simulink model "generator_of_imu"  (R2016b)
settings: Solver=ode8  StartTime=0.0  StopTime=500  FixedStep=0.01  RelTol=1e-3
undefined symbols (not defined in the file or in its folder): deg, rad, s
libraries: simulink x6, aerolibconvert2 x2, powerlib_meascontrol x2, aerolib6dof2 x1
settings Model: Creator=Utente  LastModifiedBy=Utente

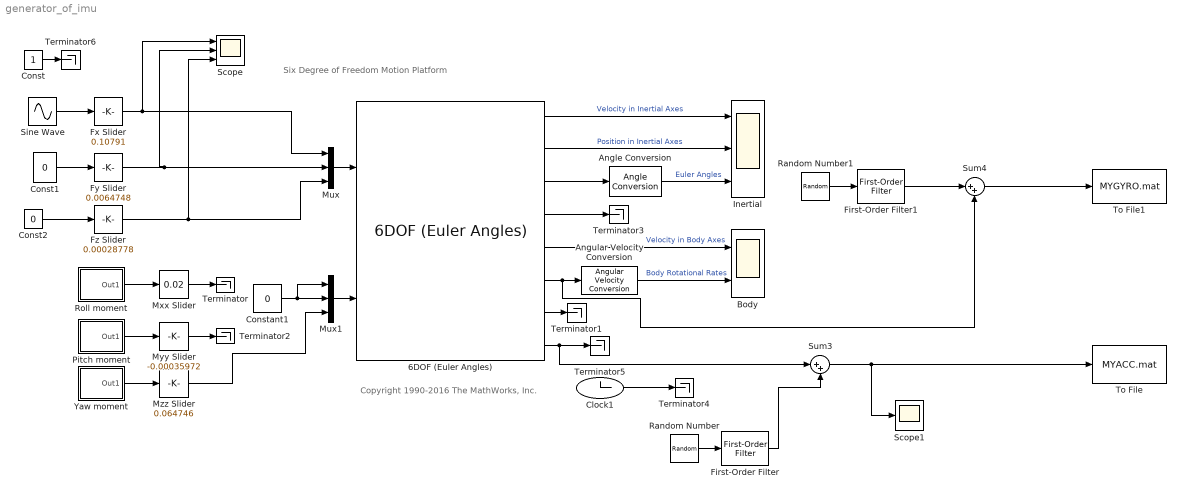
== system generator_of_imu ==
  note: Six Degree of Freedom Motion Platform
  note: Copyright 1990-2016 The MathWorks, Inc.
  6DOF (Euler Angles) : aerolib6dof2/6DOF (Euler Angles)  units=Metric (MKS)  mtype=Fixed  rep=Euler Angles  xme_0=[0 0 0]  Vm_0=[0 0 0]  eul_0=[0 0 0]  pm_0=[0 0 0]  mass_0=1.0  mass_e=0.5  mass_f=2.0  inertia=eye(3)  inertia_e=eye(3)  inertia_f=2*eye(3)  k_quat=1.0  vre_flag=on
  Angle Conversion : aerolibconvert2/Angle Conversion  IU=rad  OU=deg
  Angular Velocity Conversion : aerolibconvert2/Angular Velocity Conversion  IU=rad/s  OU=deg/s
  Body : Scope  NumInputPorts=2
  Clock1 : Clock
      settings: Decimation=100
  Const : Constant
  Const1 : Constant  Value=0
  Const2 : Constant  Value=0
  Constant1 : Constant  Value=0
  First-Order Filter : powerlib_meascontrol/Filters/First-Order Filter  FilterType=Lowpass  Tc=10  Ts=0.01  Initialize=on  Vac_Init=[0, 0, 60]  Vdc_Init=0  PlotResponse=off  FreqRange="[0,  200,  1]"
  First-Order Filter1 : powerlib_meascontrol/Filters/First-Order Filter  FilterType=Lowpass  Tc=50  Ts=0.01  Initialize=on  Vac_Init=[0, 0, 0]  Vdc_Init=0  PlotResponse=off  FreqRange="[0,  200,  1]"
  Fx Slider : simulink/Math Operations/Slider Gain  low=-1  gain=0.10791  high=1
  Fy Slider : simulink/Math Operations/Slider Gain  low=-1  gain=0.0064748  high=1
  Fz Slider : simulink/Math Operations/Slider Gain  low=-1  gain=0.00028778  high=1
  Inertial : Scope  NumInputPorts=3
  Mux : Mux  Inputs=3
  Mux1 : Mux  Inputs=3
  Mxx Slider : simulink/Math Operations/Slider Gain  low=0  gain=0.02  high=1
  Myy Slider : simulink/Math Operations/Slider Gain  low=-5  gain=-0.00035972  high=1
  Mzz Slider : simulink/Math Operations/Slider Gain  low=-3  gain=0.064746  high=3
  Pitch moment : Subsystem  mask(timed input){t=[0 3 3 4 4 5 5  7.5 7.5 8.5 8.5 9.5 9.5 10], u=[0 0  1 1 -1 -1.005 0 0 -1 -1 1 1 0 0]*3.138/2}
      mask prompts: t "time values:"; u "input values"
      mask Display: plot(t,u)
  Random Number : RandomNumber  Mean=[0;0;0]  Variance=0.09  SampleTime=0.01
  Random Number1 : RandomNumber  Mean=[0;0;0]  Variance=0.0140  SampleTime=0.01
  Roll moment : Subsystem  mask(timed input){t=[0 1 1 2 2  10], u=[1 1 -1 -.998  0 0]*3.144/2}
      mask prompts: t "time values:"; u "input values"
      mask Display: plot(t,u)
  Scope : Scope  NumInputPorts=3
  Scope1 : Scope
  Sine Wave : Sin  Amplitude=10  Frequency=10  SampleTime=0.1
  Sum3 : Sum  Inputs=|++
  Sum4 : Sum  Inputs=|++
  Terminator{,1..6} (7 alike) : Terminator
  To File : ToFile  Filename=MYACC.mat  SaveFormat=Timeseries
  To File1 : ToFile  Filename=MYGYRO.mat  SaveFormat=Timeseries
  Yaw moment : Subsystem  mask(timed input){t=[0 6 6 7 7 8 8 10], u=[0 0  -1 -1 1 1 1 1]*3.1/2}
      mask prompts: t "time values:"; u "input values"
      mask Display: plot(t,u)
  wires:
  Yaw moment/1(Out1) -> Mzz Slider/1
  Pitch moment/1(Out1) -> Myy Slider/1
  Roll moment/1(Out1) -> Mxx Slider/1
  Const2/1 -> Fz Slider/1
  Const1/1 -> Fy Slider/1
  Clock1/1 -> Terminator4/1
  Mux1/1 -> 6DOF (Euler Angles)/2
  Mzz Slider/1 -> Mux1/3
  Myy Slider/1 -> Terminator2/1
  Mxx Slider/1 -> Terminator/1
  Mux/1 -> 6DOF (Euler Angles)/1
  Fy Slider/1 -> Scope/2, Mux/2
  Fz Slider/1 -> Scope/3, Mux/3
  Fx Slider/1 -> Mux/1, Scope/1
  6DOF (Euler Angles)/4 -> Terminator3/1
  6DOF (Euler Angles)/7 -> Terminator1/1
  6DOF (Euler Angles)/3 -> Angle Conversion/1
  6DOF (Euler Angles)/5 -> Body/1  "Velocity in Body Axes"
  6DOF (Euler Angles)/1 -> Inertial/1  "Velocity in Inertial Axes"
  6DOF (Euler Angles)/2 -> Inertial/2  "Position in Inertial Axes"
  Angle Conversion/1 -> Inertial/3  "Euler Angles"
  6DOF (Euler Angles)/6 -> Sum4/2, Angular Velocity Conversion/1
  Angular Velocity Conversion/1 -> Body/2  "Body Rotational Rates"
  6DOF (Euler Angles)/8 -> Sum3/1, Terminator5/1
  Constant1/1 -> Mux1/1, Mux1/2
  Random Number/1 -> First-Order Filter/1
  First-Order Filter/1 -> Sum3/2
  Random Number1/1 -> First-Order Filter1/1
  First-Order Filter1/1 -> Sum4/1
  Sum4/1 -> To File1/1
  Const/1 -> Terminator6/1
  Sine Wave/1 -> Fx Slider/1
  Sum3/1 -> Scope1/1, To File/1

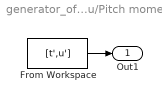
== system generator_of_imu/Pitch moment ==
  From Workspace : FromWorkspace  VariableName=[t',u']  SampleTime=0
  Out1 : Outport
  wires:
  From Workspace/1 -> Out1/1

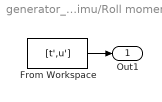
== system generator_of_imu/Roll moment ==
  From Workspace : FromWorkspace  VariableName=[t',u']  SampleTime=0
  Out1 : Outport
  wires:
  From Workspace/1 -> Out1/1

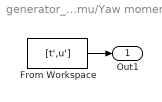
== system generator_of_imu/Yaw moment ==
  From Workspace : FromWorkspace  VariableName=[t',u']  SampleTime=0
  Out1 : Outport
  wires:
  From Workspace/1 -> Out1/1
